simulink library "xpcmeasurementcomputinglib"  (Simulink 6.0)
settings: Solver=ode45  SolverMode=SingleTasking  StartTime=0.0  StopTime=10.0  RelTol=1e-3
undefined symbols (not defined in the file or in its folder): madcbciodas, madcbpcidas, madcbpcidas1600, mctr05checks, mdacbisa, mdacbpcidas, mdacbpcidas1600, mdacbpcidda0x12, mdiocbpcipdisox, menccbcioquadcount, misa8255, mpci8255, mtccb
libraries: xpcmeasurementcomputinglib x18
(part 3 of 4)

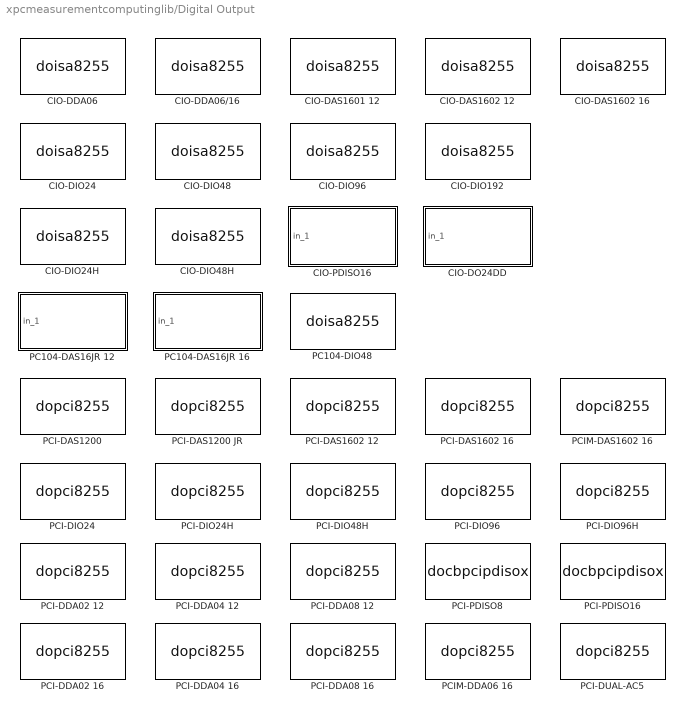
== system xpcmeasurementcomputinglib/Digital Output ==
  "CIO-DAS1601 12 " : S-Function  InitFcn=misa8255(1);  FunctionName=doisa8255  Parameters=channel, port, reset, initValue, sampletime, baseaddress, control  mask(docbciodas160112){channel=[1], port=A, reset=[1], initValue=[0], chip=1, sampletime=0.001, baseaddress=0x300}
      mask prompts: channel "Channel vector:"; reset "Reset vector:"; initValue "Initial value vector:"; sampletime "Sample time:"; baseaddress "Base address (i.e. 0xd000):"
      mask help:
      | CIO-DAS1601/12
      | ComputerBoards
      | Digital Output
      mask init:
      | baseaddress=hex2dec(baseaddress(3:end));
      | control=155;
      | boardType=16;
      | [baseaddress,control,maskdisplay,maskdescription,reset,initValue]=misa8255(2, chip, port, channel, baseaddress, reset, initValue);
      | set_param(gcb, 'MaskDisplay', maskdisplay);
      | set_param(gcb, 'MaskDescription', maskdescription);
      mask Help: helpview(fullfile(docroot, 'mapfiles', 'xpc.map'), 'ComputerBoards_CIO-DAS1601-12_DOUT')
      mask StyleString: edit,popup(A|B|C),edit,edit,popup(1),edit,edit
      mask Display: disp('CIO-DAS1601/12\nComputerBoards\nDigital Output');port_label('input',1,'1');
  "CIO-DAS1602 12 " : S-Function  InitFcn=misa8255(1);  FunctionName=doisa8255  Parameters=channel, port, reset, initValue, sampletime, baseaddress, control  mask(docbciodas160212){channel=[1], port=A, reset=[1], initValue=[0], chip=1, sampletime=0.001, baseaddress=0x300}
      mask prompts: channel "Channel vector:"; reset "Reset vector:"; initValue "Initial value vector:"; sampletime "Sample time:"; baseaddress "Base address (i.e. 0xd000):"
      mask help:
      | CIO-DAS1602/12
      | ComputerBoards
      | Digital Output
      mask init: same as xpcmeasurementcomputinglib/Digital Output/CIO-DAS1601 12 
      mask Help: helpview(fullfile(docroot, 'mapfiles', 'xpc.map'), 'ComputerBoards_CIO-DAS1602-12_DOUT')
      mask StyleString: edit,popup(A|B|C),edit,edit,popup(1),edit,edit
      mask Display: disp('CIO-DAS1602/12\nComputerBoards\nDigital Output');port_label('input',1,'1');
  "CIO-DAS1602 16 " : S-Function  InitFcn=misa8255(1);  FunctionName=doisa8255  Parameters=channel, port, reset, initValue, sampletime, baseaddress, control  mask(docbciodas160216){channel=[1], port=A, reset=[1], initValue=[0], chip=1, sampletime=0.001, baseaddress=0x300}
      mask prompts: channel "Channel vector:"; reset "Reset vector:"; initValue "Initial value vector:"; sampletime "Sample time:"; baseaddress "Base address (i.e. 0xd000):"
      mask help:
      | CIO-DAS1602/16
      | ComputerBoards
      | Digital Output
      mask init: same as xpcmeasurementcomputinglib/Digital Output/CIO-DAS1601 12 
      mask Help: helpview(fullfile(docroot, 'mapfiles', 'xpc.map'), 'ComputerBoards_CIO-DAS1602-16_DOUT')
      mask StyleString: edit,popup(A|B|C),edit,edit,popup(1),edit,edit
      mask Display: disp('CIO-DAS1602/16\nComputerBoards\nDigital Output');port_label('input',1,'1');
  "CIO-DDA06 " : S-Function  InitFcn=misa8255(1);  FunctionName=doisa8255  Parameters=channel, port, reset, initValue, sampletime, baseaddress, control  mask(docbciodda06){channel=[1], port=A, reset=[1], initValue=[0], chip=1, sampletime=0.001, baseaddress=0x300}
      mask prompts: channel "Channel vector:"; reset "Reset vector:"; initValue "Initial value vector:"; sampletime "Sample time:"; baseaddress "Base address (i.e. 0xd000):"
      mask help:
      | CIO-DDA06
      | ComputerBoards
      | Digital Output
      mask init: same as xpcmeasurementcomputinglib/Digital Output/CIO-DAS1601 12 
      mask Help: helpview(fullfile(docroot, 'mapfiles', 'xpc.map'), 'ComputerBoards_CIO-DDA06_DOUT')
      mask StyleString: edit,popup(A|B|C),edit,edit,popup(1),edit,edit
      mask Display: disp('CIO-DDA06\nComputerBoards\nDigital Output');port_label('input',1,'1');
  "CIO-DDA06/16 " : S-Function  InitFcn=misa8255(1);  FunctionName=doisa8255  Parameters=channel, port, reset, initValue, sampletime, baseaddress, control  mask(docbciodda0616){channel=[1], port=A, reset=[1], initValue=[0], chip=1, sampletime=0.001, baseaddress=0x300}
      mask prompts: channel "Channel vector:"; reset "Reset vector:"; initValue "Initial value vector:"; sampletime "Sample time:"; baseaddress "Base address (i.e. 0xd000):"
      mask help:
      | CIO-DDA06/16
      | ComputerBoards
      | Digital Output
      mask init: same as xpcmeasurementcomputinglib/Digital Output/CIO-DAS1601 12 
      mask Help: helpview(fullfile(docroot, 'mapfiles', 'xpc.map'), 'ComputerBoards_CIO-DDA06-16_DOUT')
      mask StyleString: edit,popup(A|B|C),edit,edit,popup(1),edit,edit
      mask Display: disp('CIO-DDA06/16\nComputerBoards\nDigital Output');port_label('input',1,'1');
  "CIO-DIO192 " : S-Function  InitFcn=misa8255(1);  FunctionName=doisa8255  Parameters=channel, port, reset, initValue, sampletime, baseaddress, control  mask(docbciodio192){channel=[1], port=A, reset=[1], initValue=[0], chip=1, sampletime=0.001, baseaddress=0x300}
      mask prompts: channel "Channel vector:"; reset "Reset vector:"; initValue "Initial value vector:"; sampletime "Sample time:"; baseaddress "Base address (i.e. 0xd000):"
      mask help:
      | CIO-DIO192
      | ComputerBoards
      | Digital Output
      mask init: same as xpcmeasurementcomputinglib/Digital Output/CIO-DAS1601 12 
      mask Help: helpview(fullfile(docroot, 'mapfiles', 'xpc.map'), 'ComputerBoards_CIO-DIO192_DOUT')
      mask StyleString: edit,popup(A|B|C),edit,edit,popup(1|2|3|4|5|6|7|8),edit,edit
      mask Display: disp('CIO-DIO192\nComputerBoards\nDigital Output');port_label('input',1,'1');
  "CIO-DIO24 " : S-Function  InitFcn=misa8255(1);  FunctionName=doisa8255  Parameters=channel, port, reset, initValue, sampletime, baseaddress, control  mask(docbciodio24){channel=[1], port=A, reset=[1], initValue=[0], chip=1, sampletime=0.001, baseaddress=0x300}
      mask prompts: channel "Channel vector:"; reset "Reset vector:"; initValue "Initial value vector:"; sampletime "Sample time:"; baseaddress "Base address (i.e. 0xd000):"
      mask help:
      | CIO-DIO24
      | ComputerBoards
      | Digital Output
      mask init: same as xpcmeasurementcomputinglib/Digital Output/CIO-DAS1601 12 
      mask Help: helpview(fullfile(docroot, 'mapfiles', 'xpc.map'), 'ComputerBoards_CIO-DIO24_DOUT')
      mask StyleString: edit,popup(A|B|C),edit,edit,popup(1),edit,edit
      mask Display: disp('CIO-DIO24\nComputerBoards\nDigital Output');port_label('input',1,'1');
  "CIO-DIO24H " : S-Function  InitFcn=misa8255(1);  FunctionName=doisa8255  Parameters=channel, port, reset, initValue, sampletime, baseaddress, control  mask(docbciodio24h){channel=[1], port=A, reset=[1], initValue=[0], chip=1, sampletime=0.001, baseaddress=0x300}
      mask prompts: channel "Channel vector:"; reset "Reset vector:"; initValue "Initial value vector:"; sampletime "Sample time:"; baseaddress "Base address (i.e. 0xd000):"
      mask help:
      | CIO-DIO24H
      | ComputerBoards
      | Digital Output
      mask init: same as xpcmeasurementcomputinglib/Digital Output/CIO-DAS1601 12 
      mask Help: helpview(fullfile(docroot, 'mapfiles', 'xpc.map'), 'ComputerBoards_CIO-DIO24H_DOUT')
      mask StyleString: edit,popup(A|B|C),edit,edit,popup(1),edit,edit
      mask Display: disp('CIO-DIO24H\nComputerBoards\nDigital Output');port_label('input',1,'1');
  "CIO-DIO48 " : S-Function  InitFcn=misa8255(1);  FunctionName=doisa8255  Parameters=channel, port, reset, initValue, sampletime, baseaddress, control  mask(docbciodio48){channel=[1], port=A, reset=[1], initValue=[0], chip=1, sampletime=0.001, baseaddress=0x300}
      mask prompts: channel "Channel vector:"; reset "Reset vector:"; initValue "Initial value vector:"; sampletime "Sample time:"; baseaddress "Base address (i.e. 0xd000):"
      mask help:
      | CIO-DIO48
      | ComputerBoards
      | Digital Output
      mask init: same as xpcmeasurementcomputinglib/Digital Output/CIO-DAS1601 12 
      mask Help: helpview(fullfile(docroot, 'mapfiles', 'xpc.map'), 'ComputerBoards_CIO-DIO48_DOUT')
      mask StyleString: edit,popup(A|B|C),edit,edit,popup(1|2),edit,edit
      mask Display: disp('CIO-DIO48\nComputerBoards\nDigital Output');port_label('input',1,'1');
  "CIO-DIO48H " : S-Function  InitFcn=misa8255(1);  FunctionName=doisa8255  Parameters=channel, port, reset, initValue, sampletime, baseaddress, control  mask(docbciodio48h){channel=[1], port=A, reset=[1], initValue=[0], chip=1, sampletime=0.001, baseaddress=0x300}
      mask prompts: channel "Channel vector:"; reset "Reset vector:"; initValue "Initial value vector:"; sampletime "Sample time:"; baseaddress "Base address (i.e. 0xd000):"
      mask help:
      | CIO-DIO48H
      | ComputerBoards
      | Digital Output
      mask init: same as xpcmeasurementcomputinglib/Digital Output/CIO-DAS1601 12 
      mask Help: helpview(fullfile(docroot, 'mapfiles', 'xpc.map'), 'ComputerBoards_CIO-DIO48H_DOUT')
      mask StyleString: edit,popup(A|B|C),edit,edit,popup(1|2),edit,edit
      mask Display: disp('CIO-DIO48H\nComputerBoards\nDigital Output');port_label('input',1,'1');
  "CIO-DIO96 " : S-Function  InitFcn=misa8255(1);  FunctionName=doisa8255  Parameters=channel, port, reset, initValue, sampletime, baseaddress, control  mask(docbciodio96){channel=[1], port=A, reset=[1], initValue=[0], chip=1, sampletime=0.001, baseaddress=0x300}
      mask prompts: channel "Channel vector:"; reset "Reset vector:"; initValue "Initial value vector:"; sampletime "Sample time:"; baseaddress "Base address (i.e. 0xd000):"
      mask help:
      | CIO-DIO96
      | ComputerBoards
      | Digital Output
      mask init: same as xpcmeasurementcomputinglib/Digital Output/CIO-DAS1601 12 
      mask Help: helpview(fullfile(docroot, 'mapfiles', 'xpc.map'), 'ComputerBoards_CIO-DIO96_DOUT')
      mask StyleString: edit,popup(A|B|C),edit,edit,popup(1|2|3|4),edit,edit
      mask Display: disp('CIO-DIO96\nComputerBoards\nDigital Output');port_label('input',1,'1');
  "CIO-DO24DD " : Subsystem  EnableExecutionContextPropagation=on  mask(Digital Output Module){n_channels=1, port=A, sample_time=0.001, baseaddress=0x300}
      mask prompts: n_channels "Number of channels:"; sample_time "Sample time:"; baseaddress "Base address (i.e. 0xd000):"
      mask help:
      | Computer Boards
      | CIO-DO24DD
      | Digital Output
      mask init:
      | baseaddress=hex2dec(baseaddress(3:end));
      mask Help: helpview(fullfile(docroot, 'mapfiles', 'xpc.map'), 'ComputerBoards_CIO-DO24DD_DOUT')
      mask StyleString: edit,popup(A|B|C),edit,edit
      mask Display: disp('CIO-DO24DD\nComputerBoards\nDigital Output')
  "CIO-PDISO16 " : Subsystem  EnableExecutionContextPropagation=on  mask(Digital Output Module){n_channels=1, port=1 (nearest to backplate), sample_time=0.001, baseaddress=0x300}
      mask prompts: n_channels "Number of channels:"; port "Section (connector):"; sample_time "Sample time:"; baseaddress "Base address (i.e. 0xd000):"
      mask help:
      | Computer Boards
      | CIO-PDISO16
      | Digital Output
      mask init:
      | baseaddress=hex2dec(baseaddress(3:end));
      mask Help: helpview(fullfile(docroot, 'mapfiles', 'xpc.map'), 'ComputerBoards_CIO-PDISO16_DOUT')
      mask StyleString: edit,popup(1 (nearest to backplate)|2 (farthest from backplate)),edit,edit
      mask Display: disp('CIO-PDISO16\nComputerBoards\nDigital Output')
  "PC104-DAS16JR 12 " : Subsystem  EnableExecutionContextPropagation=on  mask(Digital Output Module){n_channels=1, sample_time=0.001, baseaddress=0x300}
      mask prompts: n_channels "Number of channels:"; sample_time "Sample time:"; baseaddress "Base address (i.e. 0xd000):"
      mask help:
      | Computer Boards
      | PC104-DAS16JR/12
      | Digital Output
      mask init:
      | baseaddress=hex2dec(baseaddress(3:end));
      mask Help: helpview(fullfile(docroot, 'mapfiles', 'xpc.map'), 'ComputerBoards_PC104-DAS16JR-12_DOUT')
      mask Display: disp('PC104-DAS16JR/12\nComputerBoards\nDigital Output')
  "PC104-DAS16JR 16 " : Subsystem  EnableExecutionContextPropagation=on  mask(Digital Output Module){n_channels=1, sample_time=0.001, baseaddress=0x300}
      mask prompts: n_channels "Number of channels:"; sample_time "Sample time:"; baseaddress "Base address (i.e. 0xd000):"
      mask help:
      | Computer Boards
      | PC104-DAS16JR/16
      | Digital Output
      mask init:
      | baseaddress=hex2dec(baseaddress(3:end));
      mask Help: helpview(fullfile(docroot, 'mapfiles', 'xpc.map'), 'ComputerBoards_PC104-DAS16JR-16_DOUT')
      mask Display: disp('PC104-DAS16JR/16\nComputerBoards\nDigital Output')
  "PC104-DIO48 " : S-Function  InitFcn=misa8255(1);  FunctionName=doisa8255  Parameters=channel, port, reset, initValue, sampletime, baseaddress, control  mask(docbpc104dio48){channel=[1], port=A, reset=[1], initValue=[0], chip=1, sampletime=0.001, baseaddress=0x300}
      mask prompts: channel "Channel vector:"; reset "Reset vector:"; initValue "Initial value vector:"; sampletime "Sample time:"; baseaddress "Base address (i.e. 0xd000):"
      mask help:
      | PC104-DIO48
      | ComputerBoards
      | Digital Output
      mask init: same as xpcmeasurementcomputinglib/Digital Output/CIO-DAS1601 12 
      mask Help: helpview(fullfile(docroot, 'mapfiles', 'xpc.map'), 'ComputerBoards_PC104-DIO48_DOUT')
      mask StyleString: edit,popup(A|B|C),edit,edit,popup(1|2),edit,edit
      mask Display: disp('PC104-DIO48\nComputerBoards\nDigital Output');port_label('input',1,'1');
  "PCI-DAS1200 " : S-Function  InitFcn=mpci8255(1);  FunctionName=dopci8255  Parameters=channel, port, reset, initValue, chip, sampletime, slot, control, boardType  mask(docbpcidas1200){channel=[1], port=A, reset=[1], initValue=[0], chip=1, sampletime=0.001, slot=-1}
      mask prompts: channel "Channel vector:"; reset "Reset vector:"; initValue "Initial value vector:"; sampletime "Sample time:"; slot "PCI Slot (-1: autosearch):"
      mask help:
      | PCI-DAS1200
      | ComputerBoards
      | Digital Output
      mask init:
      | control=155;
      | [boardType,control,maskdisplay,maskdescription, reset, initValue]=mpci8255(2, chip, port, channel, slot, reset, initValue);
      | set_param(gcb, 'MaskDisplay', maskdisplay);
      | set_param(gcb, 'MaskDescription', maskdescription);
      mask Help: helpview(fullfile(docroot, 'mapfiles', 'xpc.map'), 'ComputerBoards_PCI-DAS1200_DOUT')
      mask StyleString: edit,popup(A|B|C),edit,edit,popup(1),edit,edit
      mask Display: disp('PCI-DAS1200\nComputerBoards\nDigital Output');port_label('input',1,'1');
  "PCI-DAS1200 JR " : S-Function  InitFcn=mpci8255(1);  FunctionName=dopci8255  Parameters=channel, port, reset, initValue, chip, sampletime, slot, control, boardType  mask(docbpcidas1200jr){channel=[1], port=A, reset=[1], initValue=[0], chip=1, sampletime=0.001, slot=-1}
      mask prompts: channel "Channel vector:"; reset "Reset vector:"; initValue "Initial value vector:"; sampletime "Sample time:"; slot "PCI Slot (-1: autosearch):"
      mask help:
      | PCI-DAS1200/JR
      | ComputerBoards
      | Digital Output
      mask init:
      | control=155;
      | [boardType,control,maskdisplay,maskdescription, reset, initValue]=mpci8255(2, chip, port, channel, slot, reset, initValue);
      | set_param(gcb, 'MaskDisplay', maskdisplay);
      | set_param(gcb, 'MaskDescription', maskdescription);
      mask Help: helpview(fullfile(docroot, 'mapfiles', 'xpc.map'), 'ComputerBoards_PCI-DAS1200-JR_DOUT')
      mask StyleString: edit,popup(A|B|C),edit,edit,popup(1),edit,edit
      mask Display: disp('PCI-DAS1200/JR\nComputerBoards\nDigital Output');port_label('input',1,'1');
  "PCI-DAS1602 12 " : S-Function  InitFcn=mpci8255(1);  FunctionName=dopci8255  Parameters=channel, port, reset, initValue, chip, sampletime, slot, control, boardType  mask(docbpcidas160212){channel=[1], port=A, reset=[1], initValue=[0], chip=1, sampletime=0.001, slot=-1}
      mask prompts: channel "Channel vector:"; reset "Reset vector:"; initValue "Initial value vector:"; sampletime "Sample time:"; slot "PCI Slot (-1: autosearch):"
      mask help:
      | PCI-DAS1602/12
      | ComputerBoards
      | Digital Output
      mask init: same as xpcmeasurementcomputinglib/Digital Output/PCI-DAS1200 JR 
      mask Help: helpview(fullfile(docroot, 'mapfiles', 'xpc.map'), 'ComputerBoards_PCI-DAS1602-12_DOUT')
      mask StyleString: edit,popup(A|B|C),edit,edit,popup(1),edit,edit
      mask Display: disp('PCI-DAS1602/12\nComputerBoards\nDigital Output');port_label('input',1,'1');
  "PCI-DAS1602 16 " : S-Function  InitFcn=mpci8255(1);  FunctionName=dopci8255  Parameters=channel, port, reset, initValue, chip, sampletime, slot, control, boardType  mask(docbpcidas160216){channel=[1], port=A, reset=[1], initValue=[0], chip=1, sampletime=0.001, slot=-1}
      mask prompts: channel "Channel vector:"; reset "Reset vector:"; initValue "Initial value vector:"; sampletime "Sample time:"; slot "PCI Slot (-1: autosearch):"
      mask help:
      | PCI-DAS1602/16
      | ComputerBoards
      | Digital Output
      mask init: same as xpcmeasurementcomputinglib/Digital Output/PCI-DAS1200 JR 
      mask Help: helpview(fullfile(docroot, 'mapfiles', 'xpc.map'), 'ComputerBoards_PCI-DAS1602-16_DOUT')
      mask StyleString: edit,popup(A|B|C),edit,edit,popup(1),edit,edit
      mask Display: disp('PCI-DAS1602/16\nComputerBoards\nDigital Output');port_label('input',1,'1');
  "PCI-DDA02 12 " : S-Function  InitFcn=mpci8255(1);  FunctionName=dopci8255  Parameters=channel, port, reset, initValue, chip, sampletime, slot, control, boardType  mask(docbpcidda0212){channel=[1], port=A, reset=[1], initValue=[0], chip=1, sampletime=0.001, slot=-1}
      mask prompts: channel "Channel vector:"; reset "Reset vector:"; initValue "Initial value vector:"; sampletime "Sample time:"; slot "PCI Slot (-1: autosearch):"
      mask help:
      | PCI-DDA02/12
      | ComputerBoards
      | Digital Output
      mask init: same as xpcmeasurementcomputinglib/Digital Output/PCI-DAS1200 JR 
      mask Help: helpview(fullfile(docroot, 'mapfiles', 'xpc.map'), 'ComputerBoards_PCI-DDA02-12_DOUT')
      mask StyleString: edit,popup(A|B|C),edit,edit,popup(1|2),edit,edit
      mask Display: disp('PCI-DDA02/12\nComputerBoards\nDigital Output');port_label('input',1,'1');
  "PCI-DDA02 16 " : S-Function  InitFcn=mpci8255(1);  FunctionName=dopci8255  Parameters=channel, port, reset, initValue, chip, sampletime, slot, control, boardType  mask(docbpcidda0216){channel=[1], port=A, reset=[1], initValue=[0], chip=1, sampletime=0.001, slot=-1}
      mask prompts: channel "Channel vector:"; reset "Reset vector:"; initValue "Initial value vector:"; sampletime "Sample time:"; slot "PCI Slot (-1: autosearch):"
      mask help:
      | PCI-DDA02/16
      | ComputerBoards
      | Digital Output
      mask init: same as xpcmeasurementcomputinglib/Digital Output/PCI-DAS1200 JR 
      mask Help: helpview(fullfile(docroot, 'mapfiles', 'xpc.map'), 'ComputerBoards_PCI-DDA02-16_DOUT')
      mask StyleString: edit,popup(A|B|C),edit,edit,popup(1|2),edit,edit
      mask Display: disp('PCI-DDA02/16\nComputerBoards\nDigital Output');port_label('input',1,'1');
  "PCI-DDA04 12 " : S-Function  InitFcn=mpci8255(1);  FunctionName=dopci8255  Parameters=channel, port, reset, initValue, chip, sampletime, slot, control, boardType  mask(docbpcidda0412){channel=[1], port=A, reset=[1], initValue=[0], chip=1, sampletime=0.001, slot=-1}
      mask prompts: channel "Channel vector:"; reset "Reset vector:"; initValue "Initial value vector:"; sampletime "Sample time:"; slot "PCI Slot (-1: autosearch):"
      mask help:
      | PCI-DDA04/12
      | ComputerBoards
      | Digital Output
      mask init: same as xpcmeasurementcomputinglib/Digital Output/PCI-DAS1200 JR 
      mask Help: helpview(fullfile(docroot, 'mapfiles', 'xpc.map'), 'ComputerBoards_PCI-DDA04-12_DOUT')
      mask StyleString: edit,popup(A|B|C),edit,edit,popup(1|2),edit,edit
      mask Display: disp('PCI-DDA04/12\nComputerBoards\nDigital Output');port_label('input',1,'1');
  "PCI-DDA04 16 " : S-Function  InitFcn=mpci8255(1);  FunctionName=dopci8255  Parameters=channel, port, reset, initValue, chip, sampletime, slot, control, boardType  mask(docbpcidda0416){channel=[1], port=A, reset=[1], initValue=[0], chip=1, sampletime=0.001, slot=-1}
      mask prompts: channel "Channel vector:"; reset "Reset vector:"; initValue "Initial value vector:"; sampletime "Sample time:"; slot "PCI Slot (-1: autosearch):"
      mask help:
      | PCI-DDA04/16
      | ComputerBoards
      | Digital Output
      mask init: same as xpcmeasurementcomputinglib/Digital Output/PCI-DAS1200 JR 
      mask Help: helpview(fullfile(docroot, 'mapfiles', 'xpc.map'), 'ComputerBoards_PCI-DDA04-16_DOUT')
      mask StyleString: edit,popup(A|B|C),edit,edit,popup(1|2),edit,edit
      mask Display: disp('PCI-DDA04/16\nComputerBoards\nDigital Output');port_label('input',1,'1');
  "PCI-DDA08 12 " : S-Function  InitFcn=mpci8255(1);  FunctionName=dopci8255  Parameters=channel, port, reset, initValue, chip, sampletime, slot, control, boardType  mask(docbpcidda0812){channel=[1], port=A, reset=[1], initValue=[0], chip=1, sampletime=0.001, slot=-1}
      mask prompts: channel "Channel vector:"; reset "Reset vector:"; initValue "Initial value vector:"; sampletime "Sample time:"; slot "PCI Slot (-1: autosearch):"
      mask help:
      | PCI-DDA08/12
      | ComputerBoards
      | Digital Output
      mask init: same as xpcmeasurementcomputinglib/Digital Output/PCI-DAS1200 JR 
      mask Help: helpview(fullfile(docroot, 'mapfiles', 'xpc.map'), 'ComputerBoards_PCI-DDA08-12_DOUT')
      mask StyleString: edit,popup(A|B|C),edit,edit,popup(1|2),edit,edit
      mask Display: disp('PCI-DDA08/12\nComputerBoards\nDigital Output');port_label('input',1,'1');
  "PCI-DDA08 16 " : S-Function  InitFcn=mpci8255(1);  FunctionName=dopci8255  Parameters=channel, port, reset, initValue, chip, sampletime, slot, control, boardType  mask(docbpcidda0816){channel=[1], port=A, reset=[1], initValue=[0], chip=1, sampletime=0.001, slot=-1}
      mask prompts: channel "Channel vector:"; reset "Reset vector:"; initValue "Initial value vector:"; sampletime "Sample time:"; slot "PCI Slot (-1: autosearch):"
      mask help:
      | PCI-DDA08/16
      | ComputerBoards
      | Digital Output
      mask init: same as xpcmeasurementcomputinglib/Digital Output/PCI-DAS1200 JR 
      mask Help: helpview(fullfile(docroot, 'mapfiles', 'xpc.map'), 'ComputerBoards_PCI-DDA08-16_DOUT')
      mask StyleString: edit,popup(A|B|C),edit,edit,popup(1|2),edit,edit
      mask Display: disp('PCI-DDA08/16\nComputerBoards\nDigital Output');port_label('input',1,'1');
  "PCI-DIO24 " : S-Function  InitFcn=mpci8255(1);  FunctionName=dopci8255  Parameters=channel, port, reset, initValue, chip, sampletime, slot, control, boardType  mask(docbpcidio24){channel=[1], port=A, reset=[1], initValue=[0], chip=1, sampletime=0.001, slot=-1}
      mask prompts: channel "Channel vector:"; reset "Reset vector:"; initValue "Initial value vector:"; sampletime "Sample time:"; slot "PCI Slot (-1: autosearch):"
      mask help:
      | PCI-DIO24
      | ComputerBoards
      | Digital Output
      mask init:
      | control=155;
      | [boardType,control,maskdisplay,maskdescription, reset, initValue]=mpci8255(2, chip, port, channel, slot, reset, initValue);
      | set_param(gcb, 'MaskDisplay', maskdisplay);
      | set_param(gcb, 'MaskDescription', maskdescription);
      mask Help: helpview(fullfile(docroot, 'mapfiles', 'xpc.map'), 'ComputerBoards_PCI-DIO24_DOUT')
      mask StyleString: edit,popup(A|B|C),edit,edit,popup(1),edit,edit
      mask Display: disp('PCI-DIO24\nComputerBoards\nDigital Output');port_label('input',1,'1');
  "PCI-DIO24H " : S-Function  InitFcn=mpci8255(1);  FunctionName=dopci8255  Parameters=channel, port, reset, initValue, chip, sampletime, slot, control, boardType  mask(docbpcidio24h){channel=[1], port=A, reset=[1], initValue=[0], chip=1, sampletime=0.001, slot=-1}
      mask prompts: channel "Channel vector:"; reset "Reset vector:"; initValue "Initial value vector:"; sampletime "Sample time:"; slot "PCI Slot (-1: autosearch):"
      mask help:
      | PCI-DIO24H
      | ComputerBoards
      | Digital Output
      mask init: same as xpcmeasurementcomputinglib/Digital Output/PCI-DAS1200 JR 
      mask Help: helpview(fullfile(docroot, 'mapfiles', 'xpc.map'), 'ComputerBoards_PCI-DIO24H_DOUT')
      mask StyleString: edit,popup(A|B|C),edit,edit,popup(1),edit,edit
      mask Display: disp('PCI-DIO24H\nComputerBoards\nDigital Output');port_label('input',1,'1');
  "PCI-DIO48H " : S-Function  InitFcn=mpci8255(1);  FunctionName=dopci8255  Parameters=channel, port, reset, initValue, chip, sampletime, slot, control, boardType  mask(docbpcidio48h){channel=[1], port=A, reset=[1], initValue=[0], chip=1, sampletime=0.001, slot=-1}
      mask prompts: channel "Channel vector:"; reset "Reset vector:"; initValue "Initial value vector:"; sampletime "Sample time:"; slot "PCI Slot (-1: autosearch):"
      mask help:
      | PCI-DIO48H
      | ComputerBoards
      | Digital Output
      mask init: same as xpcmeasurementcomputinglib/Digital Output/PCI-DAS1200 JR 
      mask Help: helpview(fullfile(docroot, 'mapfiles', 'xpc.map'), 'ComputerBoards_PCI-DIO48H_DOUT')
      mask StyleString: edit,popup(A|B|C),edit,edit,popup(1|2),edit,edit
      mask Display: disp('PCI-DIO48H\nComputerBoards\nDigital Output');port_label('input',1,'1');
  "PCI-DIO96 " : S-Function  InitFcn=mpci8255(1);  FunctionName=dopci8255  Parameters=channel, port, reset, initValue, chip, sampletime, slot, control, boardType  mask(docbpcidio96){channel=[1], port=A, reset=[1], initValue=[0], chip=1, sampletime=0.001, slot=-1}
      mask prompts: channel "Channel vector:"; reset "Reset vector:"; initValue "Initial value vector:"; sampletime "Sample time:"; slot "PCI Slot (-1: autosearch):"
      mask help:
      | PCI-DIO96
      | ComputerBoards
      | Digital Output
      mask init: same as xpcmeasurementcomputinglib/Digital Output/PCI-DAS1200 JR 
      mask Help: helpview(fullfile(docroot, 'mapfiles', 'xpc.map'), 'ComputerBoards_PCI-DIO96_DOUT')
      mask StyleString: edit,popup(A|B|C),edit,edit,popup(1|2|3|4),edit,edit
      mask Display: disp('PCI-DIO96\nComputerBoards\nDigital Output');port_label('input',1,'1');
  "PCI-DIO96H " : S-Function  InitFcn=mpci8255(1);  FunctionName=dopci8255  Parameters=channel, port, reset, initValue, chip, sampletime, slot, control, boardType  mask(docbpcidio96h){channel=[1], port=A, reset=[1], initValue=[0], chip=1, sampletime=0.001, slot=-1}
      mask prompts: channel "Channel vector:"; reset "Reset vector:"; initValue "Initial value vector:"; sampletime "Sample time:"; slot "PCI Slot (-1: autosearch):"
      mask help:
      | PCI-DIO96H
      | ComputerBoards
      | Digital Output
      mask init: same as xpcmeasurementcomputinglib/Digital Output/PCI-DAS1200 JR 
      mask Help: helpview(fullfile(docroot, 'mapfiles', 'xpc.map'), 'ComputerBoards_PCI-DIO96H_DOUT')
      mask StyleString: edit,popup(A|B|C),edit,edit,popup(1|2|3|4),edit,edit
      mask Display: disp('PCI-DIO96H\nComputerBoards\nDigital Output');port_label('input',1,'1');
  "PCI-DUAL-AC5 " : S-Function  InitFcn=mpci8255(1);  FunctionName=dopci8255  Parameters=channel, port, reset, initValue, chip, sampletime, slot, control, boardType  mask(docbpcidualac5){channel=[1], port=A, reset=[1], initValue=[0], chip=1, sampletime=0.001, slot=-1}
      mask prompts: channel "Channel vector:"; reset "Reset vector:"; initValue "Initial value vector:"; sampletime "Sample time:"; slot "PCI Slot (-1: autosearch):"
      mask help:
      | PCI-DUAL-AC5
      | ComputerBoards
      | Digital Output
      mask init: same as xpcmeasurementcomputinglib/Digital Output/PCI-DAS1200 JR 
      mask Help: helpview(fullfile(docroot, 'mapfiles', 'xpc.map'), 'ComputerBoards_PCI-DUAL-AC5_DOUT')
      mask StyleString: edit,popup(A|B|C),edit,edit,popup(1|2|3|4),edit,edit
      mask Display: disp('PCI-DUAL-AC5\nComputerBoards\nDigital Output');port_label('input',1,'1');
  "PCI-PDISO16 " : S-Function  InitFcn=mdiocbpcipdisox(1);  FunctionName=docbpcipdisox  Parameters=channel, port, sampletime, slot, filter, boardType  mask(docbpcipdiso16){channel=[1], filter=[0], port=A, sampletime=0.001, slot=-1}
      mask prompts: channel "Channel vector:"; filter "Filter vector:"; sampletime "Sample time:"; slot "PCI slot (-1: autosearch):"
      mask help:
      | PCI-DISO16
      | ComputerBoards
      | Digital Output
      mask init:
      | [boardType,filter,maskdisplay,maskdescription]=mdiocbpcipdisox(2, port, channel, filter, slot);
      | set_param(gcb, 'MaskDisplay', maskdisplay);
      | set_param(gcb, 'MaskDescription', maskdescription);
      mask Help: helpview(fullfile(docroot, 'mapfiles', 'xpc.map'), 'ComputerBoards_PCI-PDISO16_DOUT')
      mask StyleString: edit,edit,popup(A|B),edit,edit
      mask Display: disp('PCI-DISO16\nComputerBoards\nDigital Output');port_label('input',1,'1');
  "PCI-PDISO8 " : S-Function  InitFcn=mdiocbpcipdisox(1);  FunctionName=docbpcipdisox  Parameters=channel, port, sampletime, slot, filter, boardType  mask(docbpcipdiso8){channel=[1], filter=[0], port=A, sampletime=0.001, slot=-1}
      mask prompts: channel "Channel vector:"; filter "Filter vector:"; sampletime "Sample time:"; slot "PCI slot (-1: autosearch):"
      mask help:
      | PCI-DISO8
      | ComputerBoards
      | Digital Output
      mask init:
      | [boardType,filter,maskdisplay,maskdescription]=mdiocbpcipdisox(2, port, channel, filter, slot);
      | set_param(gcb, 'MaskDisplay', maskdisplay);
      | set_param(gcb, 'MaskDescription', maskdescription);
      mask Help: helpview(fullfile(docroot, 'mapfiles', 'xpc.map'), 'ComputerBoards_PCI-PDISO8_DOUT')
      mask StyleString: edit,edit,popup(A|B),edit,edit
      mask Display: disp('PCI-DISO8\nComputerBoards\nDigital Output');port_label('input',1,'1');
  "PCIM-DAS1602 16 " : S-Function  InitFcn=mpci8255(1);  FunctionName=dopci8255  Parameters=channel, port, reset, initValue, chip, sampletime, slot, control, boardType  mask(docbpcimdas160216){channel=[1], port=A, reset=[1], initValue=[0], chip=1, sampletime=0.001, slot=-1}
      mask prompts: channel "Channel vector:"; reset "Reset vector:"; initValue "Initial value vector:"; sampletime "Sample time:"; slot "PCI Slot (-1: autosearch):"
      mask help:
      | PCIM-DAS1602/16
      | ComputerBoards
      | Digital Output
      mask init: same as xpcmeasurementcomputinglib/Digital Output/PCI-DAS1200 JR 
      mask Help: helpview(fullfile(docroot, 'mapfiles', 'xpc.map'), 'ComputerBoards_PCIM-DAS1602-16_DOUT')
      mask StyleString: edit,popup(A|B|C),edit,edit,popup(1),edit,edit
      mask Display: disp('PCIM-DAS1602/16\nComputerBoards\nDigital Output');port_label('input',1,'1');
  "PCIM-DDA06 16 " : S-Function  InitFcn=mpci8255(1);  FunctionName=dopci8255  Parameters=channel, port, reset, initValue, chip, sampletime, slot, control, boardType  mask(docbpcimdda0616){channel=[1], port=A, reset=[1], initValue=[0], chip=1, sampletime=0.001, slot=-1}
      mask prompts: channel "Channel vector:"; reset "Reset vector:"; initValue "Initial value vector:"; sampletime "Sample time:"; slot "PCI Slot (-1: autosearch):"
      mask help:
      | PCIM-DDA06/16
      | ComputerBoards
      | Digital Output
      mask init: same as xpcmeasurementcomputinglib/Digital Output/PCI-DAS1200 JR 
      mask Help: helpview(fullfile(docroot, 'mapfiles', 'xpc.map'), 'ComputerBoards_PCIM-DDA06-16_DOUT')
      mask StyleString: edit,popup(A|B|C),edit,edit,popup(1),edit,edit
      mask Display: disp('PCIM-DDA06/16\nComputerBoards\nDigital Output');port_label('input',1,'1');

== system xpcmeasurementcomputinglib/Incremental Encoder ==
  "CIO-QUAD02 " : S-Function  InitFcn=menccbcioquadcount(0);  FunctionName=enccbcioquadcount  Parameters=convBaseAddr, channel, resetmode, polarity, mode, limit, range, speed, prescale, ts, boardtype  mask(enccbcioquadcount){channel=1, resetmode=off, polarity=Positive Index, mode=Normal, limit=5000, range=-2^23...+2^23-1, speed=1x, prescale=0, ts=0.001, baseAddr=0x300}
      mask prompts: resetmode "Index input resets counter"; polarity "Index Polarity:"; mode "Counting Mode:"; limit "Count Limit or Reset Value:"; range "Count Range:"; speed "Count Speed:"; prescale "Filter prescale factor:"; ts "Sample Time:"; baseAddr "Base Address:"
      mask help:
      | CIO-QUAD02
      | Computer Boards
      | Incremental Encoder
      mask init:
      | convBaseAddr = 0;
      | boardtype = 1;
      | [convBaseAddr] = menccbcioquadcount(1, channel , baseAddr, 0, boardtype);
      mask Help: helpview(fullfile(docroot, 'mapfiles', 'xpc.map'), 'ComputerBoards_PCI-QUAD04_Encoder')
      mask StyleString: popup(1|2|3|4),checkbox,popup(Negative Index|Positive Index),popup(Normal|Range Limit|Non-recycle|Modulo-N),edit,popup(0...2^24-1|-2^23...+2^23-1),popup(non-quadrature|1x|2x|4x),edit,edit,edit
      mask Display: text(0.05,0.75,'CIO-QUAD02','horizontalAlignment','left');text(0.05,0.5,'Comp. Boards','horizontalAlignment','left');text(0.05,0.25,'Inc. Encoder','horizontalAlignment','left');port_label('output',1,'Count')
  "CIO-QUAD04 " : S-Function  InitFcn=menccbcioquadcount(0);  FunctionName=enccbcioquadcount  Parameters=convBaseAddr, channel, resetmode, polarity, mode, limit, range, speed, prescale, ts, boardtype  mask(enccbcioquadcount){channel=1, resetmode=off, polarity=Positive Index, mode=Normal, limit=5000, range=-2^23...+2^23-1, speed=1x, prescale=0, ts=0.001, baseAddr=0x300}
      mask prompts: resetmode "Index input resets counter"; polarity "Index Polarity:"; mode "Counting Mode:"; limit "Count Limit or Reset Value:"; range "Count Range:"; speed "Count Speed:"; prescale "Filter prescale factor:"; ts "Sample Time:"; baseAddr "Base Address:"
      mask help:
      | CIO-QUAD04
      | Computer Boards
      | Incremental Encoder
      mask init:
      | convBaseAddr = 0;
      | boardtype = 2;
      | [convBaseAddr] = menccbcioquadcount(1, channel , baseAddr, 0, boardtype);
      mask Help: helpview(fullfile(docroot, 'mapfiles', 'xpc.map'), 'ComputerBoards_PCI-QUAD04_Encoder')
      mask StyleString: popup(1|2|3|4),checkbox,popup(Negative Index|Positive Index),popup(Normal|Range Limit|Non-recycle|Modulo-N),edit,popup(0...2^24-1|-2^23...+2^23-1),popup(non-quadrature|1x|2x|4x),edit,edit,edit
      mask Display: text(0.05,0.75,'CIO-QUAD04','horizontalAlignment','left');text(0.05,0.5,'Comp. Boards','horizontalAlignment','left');text(0.05,0.25,'Inc. Encoder','horizontalAlignment','left');port_label('output',1,'Count')
  "PCI-QUAD04 " : S-Function  InitFcn=menccbcioquadcount(0);  FunctionName=enccbcioquadcount  Parameters=convBaseAddr, channel, resetmode, polarity, mode, limit, range, speed, prescale, ts, boardtype  mask(enccbcioquadcount){channel=1, resetmode=off, polarity=Positive Index, mode=Normal, limit=5000, range=-2^23...+2^23-1, speed=1x, prescale=0, ts=0.001, convBaseAddr=-1}
      mask prompts: resetmode "Index input resets counter"; polarity "Index Polarity:"; mode "Counting Mode:"; limit "Count Limit or Reset Value:"; range "Count Range:"; speed "Count Speed:"; prescale "Filter prescale factor:"; ts "Sample Time:"; convBaseAddr "PCI slot (-1: autosearch):"
      mask help:
      | PCI-QUAD04
      | Computer Boards
      | Incremental Encoder
      mask init:
      | boardtype = 3;
      | menccbcioquadcount(1, channel ,'0x300', convBaseAddr, boardtype);
      mask Help: helpview(fullfile(docroot, 'mapfiles', 'xpc.map'), 'ComputerBoards_PCI-QUAD04_Encoder')
      mask StyleString: popup(1|2|3|4),checkbox,popup(Negative Index|Positive Index),popup(Normal|Range Limit|Non-recycle|Modulo-N),edit,popup(0...2^24-1|-2^23...+2^23-1),popup(non-quadrature|1x|2x|4x),edit,edit,edit
      mask Display: text(0.05,0.75,'PCI-QUAD04','horizontalAlignment','left');text(0.05,0.5,'Comp. Boards','horizontalAlignment','left');text(0.05,0.25,'Inc. Encoder','horizontalAlignment','left');port_label('output',1,'Count')

== system xpcmeasurementcomputinglib/Signal Conditioning ==

== system xpcmeasurementcomputinglib/Thermo couple ==
  "PCI-DAS-TC " : S-Function  InitFcn=mtccb(1);  FunctionName=tccbpcidastc  Parameters=resolution, average, nchannels, tctype, gain, format, cjc, sampletime, pcislot  mask(tccbpcidastc){resolution=50 Hz, average=10, nchannels=1, tctypein={'J'}, gainin=[166.7], formatin={'C'}, cjc=off, sampletime=0.1, pcislot=-1}
      mask prompts: resolution "Conversion rate (integration time):"; average "Number of samples for moving average:"; nchannels "Number of channels to be acquired (1-n):"; tctypein "Vector of thermocouple types (cell array of char):"; gainin "Vector of input gains (double array):"; formatin "Vector of temperature formats (cell array of char):"; cjc "Read and output CJC temperature"; sampletime "Sample time:"; pcislot "PCI slot (-1: autosearch):"
      mask help:
      | PCI-DAS-TC
      | ComputerBoards
      | Thermocouple Input
      mask init:
      | if resolution==3
      | 	resolution=4;
      | end
      | [tctype, gain, format, maskdisplay, maskdescription]= mtccb(2, nchannels, tctypein, gainin, formatin, cjc);
      | set_param(gcb,'MaskDescription',maskdescription);
      | set_param(gcb,'MaskDisplay',maskdisplay);
      mask Help: helpview(fullfile(docroot, 'mapfiles', 'xpc.map'), 'ComputerBoards_PCI-DAS-TC_Thermocouple')
      mask StyleString: popup(50 Hz|60 Hz|400 Hz),popup(1|2|3|4|5|6|7|8|9|10|11|12|13|14|15|16),popup(1|2|3|4|5|6|7|8|9|10|11|12|13|14|15|16),edit,edit,edit,checkbox,edit,edit
      mask Display: disp('PCI-DAS-TC\nComputerBoards\nThermocouple');port_label('output',1,'1');

== system xpcmeasurementcomputinglib/A/D/CIO-DAS16JR EXP  ==
  ADC : S-Function  FunctionName=adcbdas16jrexp  Parameters=channels, gain, admux, range, sampletime, baseaddress
  out_1 : Outport  InitialOutput=0
  wires:
  ADC/1 -> out_1/1

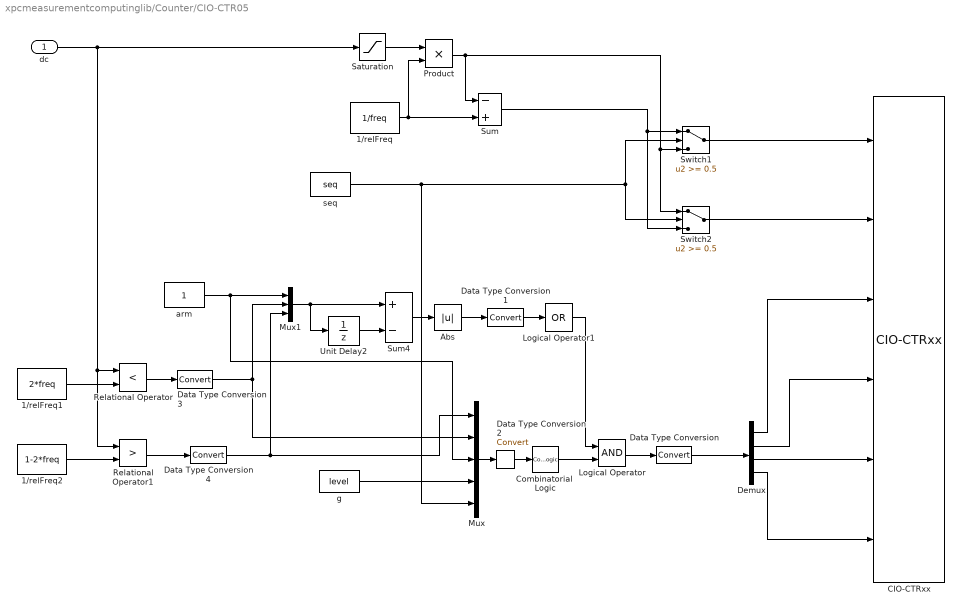
== system xpcmeasurementcomputinglib/Counter/CIO-CTR05  ==
  dc : Inport  LatchInput=off
  1/relFreq : Constant  Value=1/freq
  1/relFreq1 : Constant  Value=2*freq
  1/relFreq2 : Constant  Value=1-2*freq
  Abs : Abs  SaturateOnIntegerOverflow=on
  "CIO-CTRxx " : xpcmeasurementcomputinglib/Counter/CIO-CTRxx   mastermode=MasterMode  countermode=CounterMode  init=Init  commands=Runtime  term=Term  ts=Ts  baseAddress=baseAddress
  Combinatorial  Logic : CombinatorialLogic  TruthTable=[0,0,1,0;0,0,1,0;0,0,0,1;0,0,0,1;0,1,0,0;1,0,0,0;0,1,0,0;1,0,0,0;0,0,1,0;0,0,1,0;0,0,0,1;0,0,0,1;0,0,1,0;0,0,1,0;0,0,1,0;0,0,1,0;0,0,1,0;0,0,1,0;0,0,0,1;0,0,0,1;0,0,0,1;0,0,0,1;0,0,0,1;0,0,0,1;0,0,0,0;0,0,0,0;0,0,0,0;0,0,0,0;0,0,0,0;0,0,0,0;0,0,0,0;0,0,0,0]
  Data Type Conversion : DataTypeConversion  SaturateOnIntegerOverflow=on  RndMeth=Zero
  Data Type Conversion1 : DataTypeConversion  SaturateOnIntegerOverflow=on  RndMeth=Zero
  Data Type Conversion2 : DataTypeConversion  SaturateOnIntegerOverflow=on  RndMeth=Zero
  Data Type Conversion3 : DataTypeConversion  OutDataTypeMode=double  SaturateOnIntegerOverflow=on  RndMeth=Zero
  Data Type Conversion4 : DataTypeConversion  OutDataTypeMode=double  SaturateOnIntegerOverflow=on  RndMeth=Zero
  Demux : Demux
  Logical Operator : Logic
  Logical Operator1 : Logic  Operator=OR  Inputs=1
  Mux : Mux  Inputs=5
  Mux1 : Mux  Inputs=3
  Product : Product  SaturateOnIntegerOverflow=on  InputSameDT=on
  Relational Operator : RelationalOperator  Operator=<  InputSameDT=on
  Relational Operator1 : RelationalOperator  Operator=>  InputSameDT=on
  Saturation : Saturate  UpperLimit=1-2*freq  LowerLimit=2*freq  ZeroCross=off
  Sum : Sum  Inputs=-+  SaturateOnIntegerOverflow=on  InputSameDT=on
  Sum4 : Sum  Inputs=+-  SaturateOnIntegerOverflow=on  InputSameDT=on
  Switch1 : Switch  Threshold=0.5  InputSameDT=on
  Switch2 : Switch  Threshold=0.5  InputSameDT=on
  Unit Delay2 : UnitDelay  X0=2  SampleTime=Ts
  arm : Constant
  g : Constant  Value=level
  seq : Constant  Value=seq
  wires:
  Data Type Conversion4/1 -> Mux1/3, Mux/1
  Data Type Conversion3/1 -> Mux1/2, Mux/2
  Data Type Conversion2/1 -> Combinatorial  Logic/1
  Data Type Conversion1/1 -> Logical Operator1/1
  Data Type Conversion/1 -> Demux/1
  1/relFreq1/1 -> Relational Operator/2
  1/relFreq/1 -> Product/2, Sum/2
  Product/1 -> Sum/1, Switch1/3, Switch2/1
  1/relFreq2/1 -> Relational Operator1/2
  Relational Operator1/1 -> Data Type Conversion4/1
  Relational Operator/1 -> Data Type Conversion3/1
  Combinatorial  Logic/1 -> Logical Operator/2
  Logical Operator/1 -> Data Type Conversion/1
  Unit Delay2/1 -> Sum4/2
  Sum4/1 -> Abs/1
  Logical Operator1/1 -> Logical Operator/1
  Demux/1 -> "CIO-CTRxx "/3
  Demux/2 -> "CIO-CTRxx "/4
  Demux/3 -> "CIO-CTRxx "/5
  Demux/4 -> "CIO-CTRxx "/6
  g/1 -> Mux/4
  seq/1 -> Switch1/2, Switch2/2, Mux/5
  Sum/1 -> Switch1/1, Switch2/3
  Saturation/1 -> Product/1
  dc/1 -> Saturation/1, Relational Operator/1, Relational Operator1/1
  Mux1/1 -> Sum4/1, Unit Delay2/1
  arm/1 -> Mux1/1, Mux/3
  Abs/1 -> Data Type Conversion1/1
  Mux/1 -> Data Type Conversion2/1
  Switch1/1 -> "CIO-CTRxx "/1
  Switch2/1 -> "CIO-CTRxx "/2

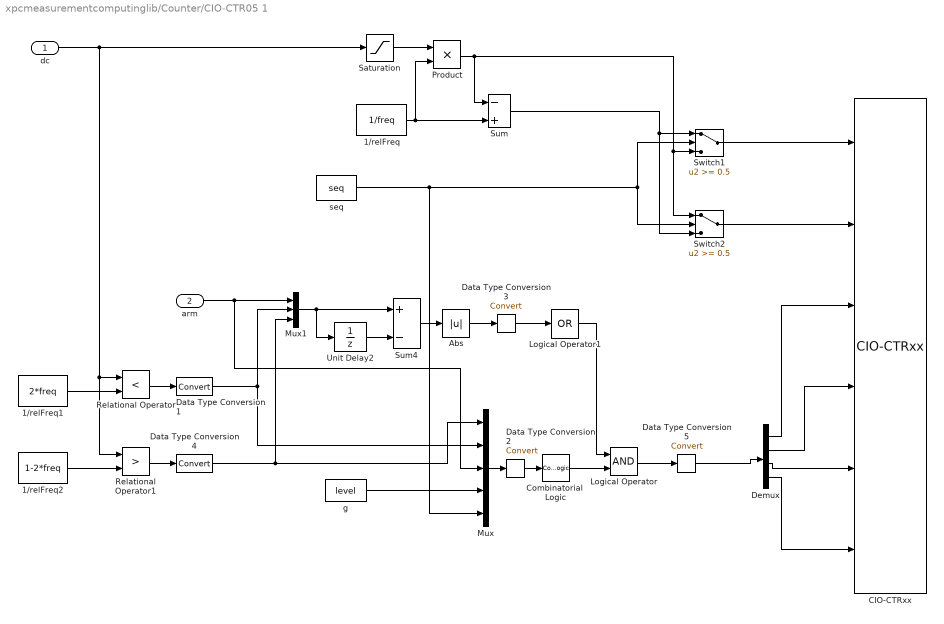
== system xpcmeasurementcomputinglib/Counter/CIO-CTR05 1 ==
  dc : Inport  LatchInput=off
  arm : Inport  Port=2  LatchInput=off
  1/relFreq : Constant  Value=1/freq
  1/relFreq1 : Constant  Value=2*freq
  1/relFreq2 : Constant  Value=1-2*freq
  Abs : Abs  SaturateOnIntegerOverflow=on
  "CIO-CTRxx " : xpcmeasurementcomputinglib/Counter/CIO-CTRxx   mastermode=MasterMode  countermode=CounterMode  init=Init  commands=Runtime  term=Term  ts=Ts  baseAddress=baseAddress
  Combinatorial  Logic : CombinatorialLogic  TruthTable=[0,0,1,0;0,0,1,0;0,0,0,1;0,0,0,1;0,1,0,0;1,0,0,0;0,1,0,0;1,0,0,0;0,0,1,0;0,0,1,0;0,0,0,1;0,0,0,1;0,0,1,0;0,0,1,0;0,0,1,0;0,0,1,0;0,0,1,0;0,0,1,0;0,0,0,1;0,0,0,1;0,0,0,1;0,0,0,1;0,0,0,1;0,0,0,1;0,0,0,0;0,0,0,0;0,0,0,0;0,0,0,0;0,0,0,0;0,0,0,0;0,0,0,0;0,0,0,0]
  Data Type Conversion1 : DataTypeConversion  OutDataTypeMode=double  SaturateOnIntegerOverflow=on  RndMeth=Zero
  Data Type Conversion2 : DataTypeConversion  SaturateOnIntegerOverflow=on  RndMeth=Zero
  Data Type Conversion3 : DataTypeConversion  SaturateOnIntegerOverflow=on  RndMeth=Zero
  Data Type Conversion4 : DataTypeConversion  OutDataTypeMode=double  SaturateOnIntegerOverflow=on  RndMeth=Zero
  Data Type Conversion5 : DataTypeConversion  SaturateOnIntegerOverflow=on  RndMeth=Zero
  Demux : Demux
  Logical Operator : Logic
  Logical Operator1 : Logic  Operator=OR  Inputs=1
  Mux : Mux  Inputs=5
  Mux1 : Mux  Inputs=3
  Product : Product  SaturateOnIntegerOverflow=on  InputSameDT=on
  Relational Operator : RelationalOperator  Operator=<  InputSameDT=on
  Relational Operator1 : RelationalOperator  Operator=>  InputSameDT=on
  Saturation : Saturate  UpperLimit=1-2*freq  LowerLimit=2*freq  ZeroCross=off
  Sum : Sum  Inputs=-+  SaturateOnIntegerOverflow=on  InputSameDT=on
  Sum4 : Sum  Inputs=+-  SaturateOnIntegerOverflow=on  InputSameDT=on
  Switch1 : Switch  Threshold=0.5  InputSameDT=on
  Switch2 : Switch  Threshold=0.5  InputSameDT=on
  Unit Delay2 : UnitDelay  X0=2  SampleTime=Ts
  g : Constant  Value=level
  seq : Constant  Value=seq
  wires:
  Data Type Conversion5/1 -> Demux/1
  Data Type Conversion3/1 -> Logical Operator1/1
  Data Type Conversion2/1 -> Combinatorial  Logic/1
  Data Type Conversion1/1 -> Mux1/2, Mux/2
  Data Type Conversion4/1 -> Mux1/3, Mux/1
  1/relFreq1/1 -> Relational Operator/2
  1/relFreq/1 -> Product/2, Sum/2
  Product/1 -> Sum/1, Switch1/3, Switch2/1
  1/relFreq2/1 -> Relational Operator1/2
  Relational Operator1/1 -> Data Type Conversion4/1
  Relational Operator/1 -> Data Type Conversion1/1
  Combinatorial  Logic/1 -> Logical Operator/2
  Logical Operator/1 -> Data Type Conversion5/1
  Unit Delay2/1 -> Sum4/2
  Sum4/1 -> Abs/1
  Logical Operator1/1 -> Logical Operator/1
  Demux/1 -> "CIO-CTRxx "/3
  Demux/2 -> "CIO-CTRxx "/4
  Demux/3 -> "CIO-CTRxx "/5
  Demux/4 -> "CIO-CTRxx "/6
  g/1 -> Mux/4
  seq/1 -> Switch1/2, Switch2/2, Mux/5
  Sum/1 -> Switch1/1, Switch2/3
  Saturation/1 -> Product/1
  dc/1 -> Saturation/1, Relational Operator/1, Relational Operator1/1
  Mux1/1 -> Sum4/1, Unit Delay2/1
  arm/1 -> Mux1/1, Mux/3
  Abs/1 -> Data Type Conversion3/1
  Mux/1 -> Data Type Conversion2/1
  Switch1/1 -> "CIO-CTRxx "/1
  Switch2/1 -> "CIO-CTRxx "/2

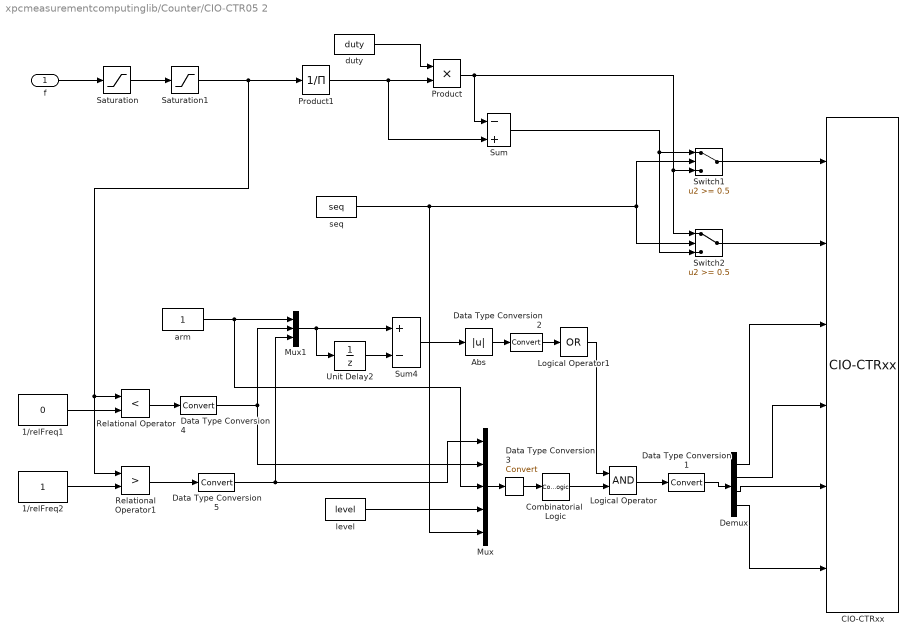
== system xpcmeasurementcomputinglib/Counter/CIO-CTR05 2 ==
  f : Inport  LatchInput=off
  1/relFreq1 : Constant  Value=0
  1/relFreq2 : Constant
  Abs : Abs  SaturateOnIntegerOverflow=on
  "CIO-CTRxx " : xpcmeasurementcomputinglib/Counter/CIO-CTRxx   mastermode=MasterMode  countermode=CounterMode  init=Init  commands=Runtime  term=Term  ts=Ts  baseAddress=baseAddress
  Combinatorial  Logic : CombinatorialLogic  TruthTable=[0,0,1,0;0,0,1,0;0,0,0,1;0,0,0,1;0,1,0,0;1,0,0,0;0,1,0,0;1,0,0,0;0,0,1,0;0,0,1,0;0,0,0,1;0,0,0,1;0,0,1,0;0,0,1,0;0,0,1,0;0,0,1,0;0,0,1,0;0,0,1,0;0,0,0,1;0,0,0,1;0,0,0,1;0,0,0,1;0,0,0,1;0,0,0,1;0,0,0,0;0,0,0,0;0,0,0,0;0,0,0,0;0,0,0,0;0,0,0,0;0,0,0,0;0,0,0,0]
  Data Type Conversion1 : DataTypeConversion  SaturateOnIntegerOverflow=on  RndMeth=Zero
  Data Type Conversion2 : DataTypeConversion  SaturateOnIntegerOverflow=on  RndMeth=Zero
  Data Type Conversion3 : DataTypeConversion  SaturateOnIntegerOverflow=on  RndMeth=Zero
  Data Type Conversion4 : DataTypeConversion  OutDataTypeMode=double  SaturateOnIntegerOverflow=on  RndMeth=Zero
  Data Type Conversion5 : DataTypeConversion  OutDataTypeMode=double  SaturateOnIntegerOverflow=on  RndMeth=Zero
  Demux : Demux
  Logical Operator : Logic
  Logical Operator1 : Logic  Operator=OR  Inputs=1
  Mux : Mux  Inputs=5
  Mux1 : Mux  Inputs=3
  Product : Product  SaturateOnIntegerOverflow=on  InputSameDT=on
  Product1 : Product  Inputs=/  SaturateOnIntegerOverflow=on  InputSameDT=on
  Relational Operator : RelationalOperator  Operator=<  InputSameDT=on
  Relational Operator1 : RelationalOperator  Operator=>  InputSameDT=on
  Saturation : Saturate  UpperLimit=duty/2  LowerLimit=duty/(2^16-1)  ZeroCross=off
  Saturation1 : Saturate  UpperLimit=(1-duty)/2  LowerLimit=(1-duty)/(2^16-1)  ZeroCross=off
  Sum : Sum  Inputs=-+  SaturateOnIntegerOverflow=on  InputSameDT=on
  Sum4 : Sum  Inputs=+-  SaturateOnIntegerOverflow=on  InputSameDT=on
  Switch1 : Switch  Threshold=0.5  InputSameDT=on
  Switch2 : Switch  Threshold=0.5  InputSameDT=on
  Unit Delay2 : UnitDelay  X0=2  SampleTime=Ts
  arm : Constant
  duty : Constant  Value=duty
  level : Constant  Value=level
  seq : Constant  Value=seq
  wires:
  Data Type Conversion5/1 -> Mux1/3, Mux/1
  Data Type Conversion4/1 -> Mux1/2, Mux/2
  Data Type Conversion3/1 -> Combinatorial  Logic/1
  Data Type Conversion2/1 -> Logical Operator1/1
  Data Type Conversion1/1 -> Demux/1
  1/relFreq1/1 -> Relational Operator/2
  Product/1 -> Sum/1, Switch1/3, Switch2/1
  1/relFreq2/1 -> Relational Operator1/2
  Relational Operator1/1 -> Data Type Conversion5/1
  Relational Operator/1 -> Data Type Conversion4/1
  Combinatorial  Logic/1 -> Logical Operator/2
  Logical Operator/1 -> Data Type Conversion1/1
  Unit Delay2/1 -> Sum4/2
  Sum4/1 -> Abs/1
  Logical Operator1/1 -> Logical Operator/1
  Demux/1 -> "CIO-CTRxx "/3
  Demux/2 -> "CIO-CTRxx "/4
  Demux/3 -> "CIO-CTRxx "/5
  Demux/4 -> "CIO-CTRxx "/6
  level/1 -> Mux/4
  Switch1/1 -> "CIO-CTRxx "/1
  Switch2/1 -> "CIO-CTRxx "/2
  seq/1 -> Switch1/2, Switch2/2, Mux/5
  Sum/1 -> Switch1/1, Switch2/3
  Saturation/1 -> Saturation1/1
  f/1 -> Saturation/1
  Mux1/1 -> Sum4/1, Unit Delay2/1
  arm/1 -> Mux1/1, Mux/3
  Abs/1 -> Data Type Conversion2/1
  Mux/1 -> Data Type Conversion3/1
  Saturation1/1 -> Product1/1, Relational Operator1/1, Relational Operator/1
  duty/1 -> Product/1
  Product1/1 -> Product/2, Sum/2
